simulink model "selecting_elements_from_a_1D_array"  (R2016b)
settings: Solver=ode4  StartTime=0.0  StopTime=9  FixedStep=1  RelTol=1e-3
settings Model: Creator=mbatu  LastModifiedBy=mbatu

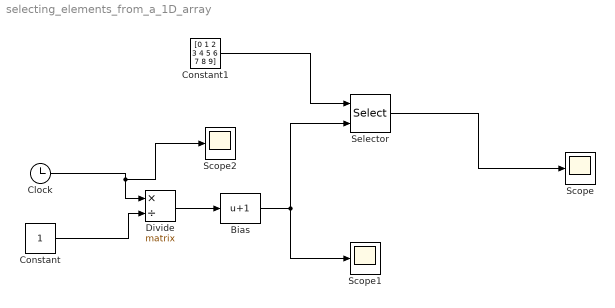
== system selecting_elements_from_a_1D_array ==
  Bias : Bias  Bias=1
  Clock : Clock
  Constant : Constant
  Constant1 : Constant  Value=[0 1 2 3 4 5 6 7 8 9]  OutDataTypeStr=double  SampleTime=-1
  Divide : Product  Inputs=*/  Multiplication=Matrix(*)
  Scope : Scope
  Scope1 : Scope
  Scope2 : Scope
  Selector : Selector  IndexOptions=Index vector (port)  Indices=[1 3]  OutputSizes=1
  wires:
  Constant/1 -> Divide/2
  Constant1/1 -> Selector/1
  Divide/1 -> Bias/1
  Clock/1 -> Scope2/1, Divide/1
  Bias/1 -> Selector/2, Scope1/1
  Selector/1 -> Scope/1
